simulink model "SimulinkModel2"  (R2020a)
settings: Solver=VariableStepAuto  StartTime=0.0  StopTime=.5  RelTol=1e-3
libraries: powerlib x21
settings Model: Creator=TommyBoy  LastModifiedBy=TommyBoy

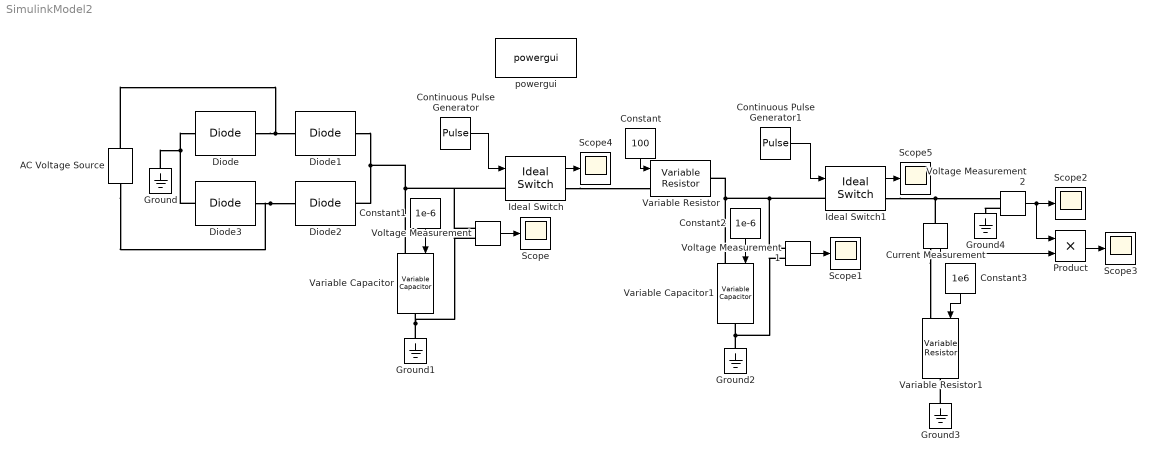
== system SimulinkModel2 ==
  AC Voltage Source : powerlib/Electrical Sources/AC Voltage Source  Amplitude=100  Phase=0  Frequency=60  SampleTime=0  Measurements=None  BusType=swing  Pref=10e3  Qref=0  Qmin=-inf  Qmax=+inf
  Constant : Constant  Value=100
  Constant1 : Constant  Value=1e-6
  Constant2 : Constant  Value=1e-6
  Constant3 : Constant  Value=1e6
  Continuous Pulse Generator : DiscretePulseGenerator  PulseType=Time based  Period=50e-3  PulseWidth=50
  Continuous Pulse Generator1 : DiscretePulseGenerator  PulseType=Time based  Period=50e-3  PulseWidth=50  PhaseDelay=25e-3
  Current Measurement : powerlib/Measurements/Current Measurement  PhasorSimulation=off  OutputType=Complex  PSBequivalent=0
  Diode{,1..3} (4 alike) : powerlib/Power Electronics/Diode  Ron=0.001  Lon=0  Vf=0.8  IC=0  UseSnubber=0  Rs=500  Cs=250e-9  Measurements=off
  Ground{,1..4} (5 alike) : powerlib/Elements/Ground  LConnTagsString=a
  Ideal Switch : powerlib/Power Electronics/Ideal Switch  Ron=0.001  Lon=0  IC=0  Rs=1e5  Cs=inf  Measurements=on
  Ideal Switch1 : powerlib/Power Electronics/Ideal Switch  Ron=0.001  Lon=0  IC=0  Rs=1e5  Cs=inf  Measurements=on
  Product : Product
  Scope{,1..5} (6 alike) : Scope
  Variable Capacitor : powerlib/Elements/Variable Capacitor  methode=Backward Euler  Cabsmin=1e-9  Initialize=off  vC0=0  C0=1e-6  iC0=2.073e-16
      settings: SourceProductBaseCode=PS
  Variable Capacitor1 : powerlib/Elements/Variable Capacitor  methode=Backward Euler  Cabsmin=1e-9  Initialize=off  vC0=0  C0=1e-6  iC0=0
      settings: SourceProductBaseCode=PS
  Variable Resistor : powerlib/Elements/Variable Resistor  Rabsmin=100
      settings: SourceProductBaseCode=PS
  Variable Resistor1 : powerlib/Elements/Variable Resistor  Rabsmin=1e6
      settings: SourceProductBaseCode=PS
  Voltage Measurement : powerlib/Measurements/Voltage Measurement  PhasorSimulation=off  OutputType=Complex  PSBequivalent=0
  Voltage Measurement1 : powerlib/Measurements/Voltage Measurement  PhasorSimulation=off  OutputType=Complex  PSBequivalent=0
  Voltage Measurement2 : powerlib/Measurements/Voltage Measurement  PhasorSimulation=off  OutputType=Complex  PSBequivalent=0
  powergui : powerlib/powergui  Priority=1  SimulationMode=Discrete  SampleTime=0.001  frequency=60  Iterations=50  frequencyindice=60  Pbase=100e6  ErrMax=1e-4  UnitsV=kV  UnitsW=MW  buscounter=0  FunctionMessages=off  echomessages=off  EnableUseOfTLC=off  CurrentSourceSwitches=off  DisableSnubberDevices=off  DisableRonSwitches=off  DisableVfSwitches=off  DisplayEquations=off  AutomaticDiscreteSolvers=off  SolverType=Tustin/Backward Euler (TBE)  Interpol=off  ExternalGateDelay=off  methode=off  Ts=100  x0status=blocks  SPID=on  SwTol=0  HookPort=off  NonlinearTolerance=1e-4  nMaxIteration=100  ContinueOnMaxIteration=off  RestoreLinks=warning  ResistiveCurrentMeasurement=off  Frange=[0:2:500]  Ylog=off  Xlog=on  ShowGrid=off  save=off  variable=ZData  structure=0  ZoomFFT=off  StartTime=0.0  cycles=1  DisplayStyle=1  fundamental=60  FreqAxis=off  MaxFrequency=1000  frequencyindicesteady=1  RmsSteady=1  display=off
  wires:
  Voltage Measurement/1 -> Scope/1
  Continuous Pulse Generator/1 -> Ideal Switch/1
  Voltage Measurement1/1 -> Scope1/1
  Continuous Pulse Generator1/1 -> Ideal Switch1/1
  Constant/1 -> Variable Resistor/1
  Constant1/1 -> Variable Capacitor/1
  Constant2/1 -> Variable Capacitor1/1
  Constant3/1 -> Variable Resistor1/1
  Current Measurement/1 -> Product/2
  Voltage Measurement2/1 -> Product/1, Scope2/1
  Product/1 -> Scope3/1
  Ideal Switch/1 -> Scope4/1
  Ideal Switch1/1 -> Scope5/1
  connections:
  Diode3/RConn1 -- Diode2/LConn1 -- AC Voltage Source/LConn1
  Diode3/LConn1 -- Ground/LConn1 -- Diode/LConn1
  Diode/RConn1 -- Diode1/LConn1 -- AC Voltage Source/RConn1
  Diode1/RConn1 -- Ideal Switch/LConn1 -- Voltage Measurement/LConn1 -- Variable Capacitor/LConn1 -- Diode2/RConn1
  Ground1/LConn1 -- Variable Capacitor/RConn1 -- Voltage Measurement/LConn2
  Ideal Switch/RConn1 -- Variable Resistor/LConn1
  Voltage Measurement1/LConn1 -- Ideal Switch1/LConn1 -- Variable Resistor/RConn1 -- Variable Capacitor1/LConn1
  Ground2/LConn1 -- Voltage Measurement1/LConn2 -- Variable Capacitor1/RConn1
  Ideal Switch1/RConn1 -- Current Measurement/LConn1 -- Voltage Measurement2/LConn1
  Ground3/LConn1 -- Variable Resistor1/RConn1
  Current Measurement/RConn1 -- Variable Resistor1/LConn1
  Voltage Measurement2/LConn2 -- Ground4/LConn1
